simulink library "INT_Clth_DD"  (R2016b)
settings: Solver=VariableStepAuto  StartTime=0.0  StopTime=10.0  RelTol=1e-3
settings Model: Creator=Administrator  LastModifiedBy=Administrator

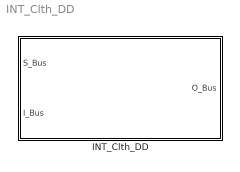
== system INT_Clth_DD ==
  INT_Clth_DD : Subsystem

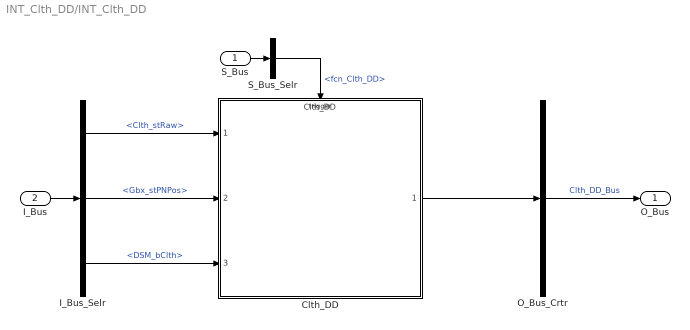
== system INT_Clth_DD/INT_Clth_DD ==
  S_Bus : Inport
  I_Bus : Inport  Port=2
  Clth_DD : ModelReference  ModelNameDialog=Clth_DD  SimulationMode=Normal  ModelReferenceVersion=1.9  TriggerPortName=function  TriggerPortTriggerType=function-call  TriggerPortStatesWhenEnabling=held
  I_Bus_Selr : BusSelector  OutputSignals=Clth_stRaw,Gbx_stPNPos,DSM_bClth
  O_Bus_Crtr : BusCreator  Inputs=1
  S_Bus_Selr : BusSelector  OutputSignals=fcn_Clth_DD
  O_Bus : Outport
  wires:
  S_Bus_Selr/1 -> Clth_DD/Trigger  "<fcn_Clth_DD>"
  S_Bus/1 -> S_Bus_Selr/1
  I_Bus/1 -> I_Bus_Selr/1
  I_Bus_Selr/1 -> Clth_DD/1  "<Clth_stRaw>"
  I_Bus_Selr/2 -> Clth_DD/2  "<Gbx_stPNPos>"
  I_Bus_Selr/3 -> Clth_DD/3  "<DSM_bClth>"
  O_Bus_Crtr/1 -> O_Bus/1  "Clth_DD_Bus"
  Clth_DD/1 -> O_Bus_Crtr/1
